simulink model "node23_case_10kV_withLoad_v2"  (R2022b)
settings: Solver=VariableStepAuto  StartTime=0.0  StopTime=10  FixedStep=1e-6  RelTol=1e-5
InitFcn:
  | sw=5;
  | Lf=1.75e-3+3.5e-3;
  | %Lf=3.5e-3;
  | %Cf=2e-4;
  | f=10;
  | Cf=15e-6;
  | % L=1.75e-3/2;
  | % X=100*pi*L;
  | % R=2*X;
  | R=0.25;X=R/0.66;
  | L=X/100/pi;
  | Z=sqrt(R^2+X^2);
  | f = 30;
  | kp1=10;
  | ki1=100;
  | kp4=20;
  | ki4=100;
  | kp16=20;
  | ki16=100;
  | % 负载参数
  | R1L=0;
  | X1L=0;
  | R2L=652.4467;
  | X2L=276.0351;
  | R3L=804.5741;
  | X3L=256.7790;
  | R4L=760.9867;
  | X4L=234.6376;
  | R5L=818.7384;
  | X5L=266.9799;
  | R6L=671.1329;
  | X6L=170.1801;
  | R7L=883.7621;
  | X7L=178.8663;
  | R8L=388.3725;
  | X8L=158.3040;
  | R9L=817.4819;
  | X9L=268.6933;
  | R10L=849.4733;
  | X10L=254.8420;
  | R11L=407.8415;
  | X11L=165.8504;
  | R12L=NaN;  % Bus 12 无 R、X 数据，用 NaN 标记
  | X12L=NaN;
  | R13L=751.2339;
  | X13L=329.8428;
  | R14L=294.0393;
  | X14L=141.6929;
  | R15L=761.9027;
  | X15L=284.3908;
  | R16L=740.4040;
  | X16L=318.2438;
  | R17L=674.5784;
  | X17L=316.4689;
  | R18L=776.7449;
  | X18L=316.6080;
  | R19L=766.0423;
  | X19L=335.7994;
  | R20L=746.0545;
  | X20L=344.3329;
  | ... (+266 lines)
libraries: spsSeriesRLCBranchLib x210, slpidlib x45, spsControlledVoltageSourceLib x30, spsThreePhaseVIMeasurementLib x24, spsPower3phInstantaneousLib x13, spsAlphaBetaZerotoabcLib x9, spsCurrentMeasurementLib x6, spsGroundLib x2, spspowerguiLib x1
(part 6 of 8)

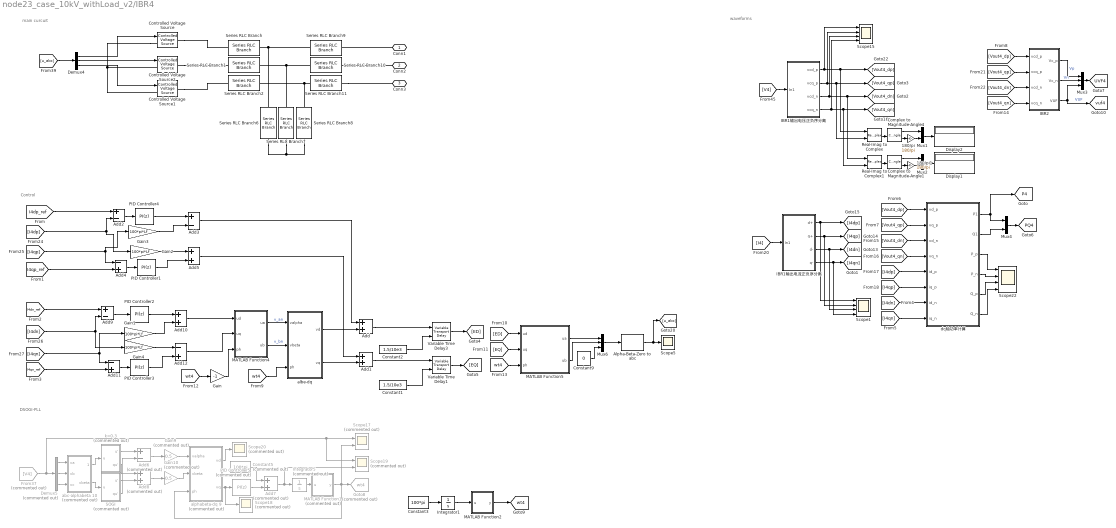
== system node23_case_10kV_withLoad_v2/IBR4 ==
  note: waveforms
  note: Control
  note: main curcuit
  note: DSOGI-PLL
  180/pi : Gain  Gain=180/pi
  180/pi1 : Gain  Gain=180/pi
  Add{,1,5,10} (4 alike) : Sum
  Add11 : Sum  Inputs=-+
  Add12 : Sum  Inputs=-+
  Add2 : Sum  Inputs=+-
  Add3 : Sum  Inputs=+-
  Add4 : Sum  Inputs=-+
  Add6 : Sum  Commented=on  Inputs=+-
  Add7 : Sum  Commented=on
  Add8 : Sum  Commented=on
  Add9 : Sum  Inputs=+-
  Alpha-Beta-Zero to abc : spsAlphaBetaZerotoabcLib/Alpha-Beta-Zero to abc
      settings: LibrarySourceBlock=|
      | sps_lib/Control/Alpha-Beta-Zero
      | to abc
  Complex to Magnitude-Angle1 : ComplexToMagnitudeAngle
  Complex to Magnitude-Angle4 : ComplexToMagnitudeAngle
  Constant1 : Constant  Value=1.5/10e3
  Constant2 : Constant  Value=1.5/10e3
  Constant3 : Constant  Value=100*pi
  Constant5 : Constant  Commented=on  Value=100*pi
  Constant9 : Constant  Value=0
  Controlled Voltage Source : spsControlledVoltageSourceLib/Controlled Voltage Source  Initialize=on  Source_Type=AC  Amplitude=0  Phase=0  Frequency=0  Measurements=None
  Controlled Voltage Source1 : spsControlledVoltageSourceLib/Controlled Voltage Source  Initialize=on  Source_Type=AC  Amplitude=0  Phase=0  Frequency=0  Measurements=None
  Controlled Voltage Source2 : spsControlledVoltageSourceLib/Controlled Voltage Source  Initialize=on  Source_Type=AC  Amplitude=0  Phase=0  Frequency=0  Measurements=None
  Demux4 : Demux  Outputs=3
  Demux5 : Demux  Commented=on  Outputs=3
  Display1 : Display
  Display2 : Display
  From37 : From  Commented=on  GotoTag=V4  TagVisibility=global
  Gain : Gain  Gain=-1
  Gain{1..4} (4 alike) : Gain  Gain=100*pi*Lf
  Gain10 : Gain  Commented=on  Gain=0.5
  Gain9 : Gain  Commented=on  Gain=0.5
  Goto8 : Goto  Commented=on  GotoTag=wt4  TagVisibility=global
  IBR1输出电压正负序分离 : Subsystem
  IBR1输出电流正负序分离 : Subsystem
  IBR2 : MATLAB Function  TreatAsAtomicUnit=on
  Integrator1 : Integrator
  Integrator5 : Integrator  Commented=on
  MATLAB Function1 : MATLAB Function  Commented=on  TreatAsAtomicUnit=on
  MATLAB Function2 : MATLAB Function  TreatAsAtomicUnit=on
  MATLAB Function4 : MATLAB Function  TreatAsAtomicUnit=on
  MATLAB Function5 : MATLAB Function  TreatAsAtomicUnit=on
  Mux1 : Mux  Inputs=2
  Mux2 : Mux  Inputs=2
  Mux3 : Mux  Inputs=3
  Mux4 : Mux  Inputs=2
  Mux6 : Mux  Inputs=3
  PID Controller{1..4} (4 alike) : slpidlib/PID Controller  Controller=PI  Form=Parallel  TimeDomain=Discrete-time  UseExternalTs=off  SampleTime=-1  IntegratorMethod=Forward Euler  FilterMethod=Forward Euler  ControllerParametersSource=internal  P=kp4  I=ki4  UseKiTs=off  D=0  N=100  UseFilter=on  TunerSelectOption=Transfer Function Based (PID Tuner App)  InitialConditionSource=internal  InitialConditionForIntegrator=0  InitialConditionForFilter=0  DifferentiatorICPrevScaledInput=0  ExternalReset=none  TrackingMode=off  Kt=1  LimitOutput=off  SatLimitsSource=internal  UpperSaturationLimit=5  LowerSaturationLimit=-5  LinearizeAsGain=on  AntiWindupMode=none  Kb=1  LimitIntegrator=off  UpperIntegratorSaturationLimit=inf  LowerIntegratorSaturationLimit=-inf  POutMin=[]  POutMax=[]  IOutMin=[]  IOutMax=[]  DOutMin=[]  DOutMax=[]  NOutMin=[]  NOutMax=[]  SumOutMin=[]  SumOutMax=[]  SaturationOutMin=[]  SaturationOutMax=[]  PParamMin=[]  PParamMax=[]  IParamMin=[]  IParamMax=[]  DParamMin=[]  DParamMax=[]  NParamMin=[]  NParamMax=[]  KbParamMin=[]  KbParamMax=[]  KtParamMin=[]  KtParamMax=[]  KbOutMin=[]  KbOutMax=[]  KtOutMin=[]  KtOutMax=[]  IntegratorOutMin=[]  IntegratorOutMax=[]  FilterOutMin=[]  FilterOutMax=[]  SumI1OutMin=[]  SumI1OutMax=[]  SumI2OutMin=[]  SumI2OutMax=[]  SumI3OutMin=[]  SumI3OutMax=[]  SumI4OutMin=[]  SumI4OutMax=[]  SumDOutMin=[]  SumDOutMax=[]  DifferentiatorOutMin=[]  DifferentiatorOutMax=[]  FilterDiffOutCoefMin=[]  FilterDiffOutCoefMax=[]  ReciprocalOutMin=[]  ReciprocalOutMax=[]  SumDenOutMin=[]  SumDenOutMax=[]  SumNumOutMin=[]  SumNumOutMax=[]  DivideOutMin=[]  DivideOutMax=[]  UdiffTsProdOutMin=[]  UdiffTsProdOutMax=[]  NTsProdOutMin=[]  NTsProdOutMax=[]  UintegralTsProdOutMin=[]  UintegralTsProdOutMax=[]  UngainTsProdOutMin=[]  UngainTsProdOutMax=[]  ClampingZeroOutDataTypeStr=Inherit: Inherit via back propagation  ClampingZeroOutMin=[]  ClampingZeroOutMax=[]  FilterDenConstantOutDataTypeStr=Inherit: Inherit via back propagation  FilterDenConstantOutMin=[]  FilterDenConstantOutMax=[]  PCopyOutDataTypeStr=Inherit: Inherit via back propagation  PCopyOutMin=[]  PCopyOutMax=[]  NCopyOutDataTypeStr=Inherit: Inherit via back propagation  NCopyOutMin=[]  NCopyOutMax=[]  IntegratorContinuousStateAttributes=''  IntegratorStateMustResolveToSignalObject=off  IntegratorRTWStateStorageClass=Auto  FilterContinuousStateAttributes=''  FilterStateMustResolveToSignalObject=off  FilterRTWStateStorageClass=Auto  ParallelPVariant=InternalParameters  IdealPVariant=Disabled  IVariant=InternalParameters  DVariant=Disabled  IntegratorVariant=Discrete  SatVariant=Disabled  AWVariant=Passthrough  PCopyVariant=Disabled  TRVariant=Disabled  FdbkBlocksVariant=Forward  IdealPFdbkVariant=Disabled  SatFdbkVariant=Disabled  DerivativeFilterVariant=Disabled  NVariant=Disabled  NCopyVariant=Disabled_SignalSpec  FilterICVariant=Disabled  IntegratorICVariant=InternalICs  ExternalResetVariant=Disabled  TRSumVariant=Passthrough  SumFdbkVariant=Disabled  SumVariant=Sum_PI  TsampFilterVariant=InternalTs  TsampNgainVariant=Passthrough  TsampIntegralVariant=Passthrough  ExternalSaturationOutDataTypeStr=Inherit: Same as second input
  PID Controller5 : slpidlib/PID Controller  Commented=on  Controller=PI  Form=Parallel  TimeDomain=Discrete-time  UseExternalTs=off  SampleTime=-1  IntegratorMethod=Forward Euler  FilterMethod=Forward Euler  ControllerParametersSource=internal  P=1  I=3  UseKiTs=off  D=0  N=100  UseFilter=on  TunerSelectOption=Transfer Function Based (PID Tuner App)  InitialConditionSource=internal  InitialConditionForIntegrator=0  InitialConditionForFilter=0  DifferentiatorICPrevScaledInput=0  ExternalReset=none  TrackingMode=off  Kt=1  LimitOutput=off  SatLimitsSource=internal  UpperSaturationLimit=inf  LowerSaturationLimit=-inf  LinearizeAsGain=on  AntiWindupMode=none  Kb=1  LimitIntegrator=off  UpperIntegratorSaturationLimit=inf  LowerIntegratorSaturationLimit=-inf  POutMin=[]  POutMax=[]  IOutMin=[]  IOutMax=[]  DOutMin=[]  DOutMax=[]  NOutMin=[]  NOutMax=[]  SumOutMin=[]  SumOutMax=[]  SaturationOutMin=[]  SaturationOutMax=[]  PParamMin=[]  PParamMax=[]  IParamMin=[]  IParamMax=[]  DParamMin=[]  DParamMax=[]  NParamMin=[]  NParamMax=[]  KbParamMin=[]  KbParamMax=[]  KtParamMin=[]  KtParamMax=[]  KbOutMin=[]  KbOutMax=[]  KtOutMin=[]  KtOutMax=[]  IntegratorOutMin=[]  IntegratorOutMax=[]  FilterOutMin=[]  FilterOutMax=[]  SumI1OutMin=[]  SumI1OutMax=[]  SumI2OutMin=[]  SumI2OutMax=[]  SumI3OutMin=[]  SumI3OutMax=[]  SumI4OutMin=[]  SumI4OutMax=[]  SumDOutMin=[]  SumDOutMax=[]  DifferentiatorOutMin=[]  DifferentiatorOutMax=[]  FilterDiffOutCoefMin=[]  FilterDiffOutCoefMax=[]  ReciprocalOutMin=[]  ReciprocalOutMax=[]  SumDenOutMin=[]  SumDenOutMax=[]  SumNumOutMin=[]  SumNumOutMax=[]  DivideOutMin=[]  DivideOutMax=[]  UdiffTsProdOutMin=[]  UdiffTsProdOutMax=[]  NTsProdOutMin=[]  NTsProdOutMax=[]  UintegralTsProdOutMin=[]  UintegralTsProdOutMax=[]  UngainTsProdOutMin=[]  UngainTsProdOutMax=[]  ClampingZeroOutDataTypeStr=Inherit: Inherit via back propagation  ClampingZeroOutMin=[]  ClampingZeroOutMax=[]  FilterDenConstantOutDataTypeStr=Inherit: Inherit via back propagation  FilterDenConstantOutMin=[]  FilterDenConstantOutMax=[]  PCopyOutDataTypeStr=Inherit: Inherit via back propagation  PCopyOutMin=[]  PCopyOutMax=[]  NCopyOutDataTypeStr=Inherit: Inherit via back propagation  NCopyOutMin=[]  NCopyOutMax=[]  IntegratorContinuousStateAttributes=''  IntegratorStateMustResolveToSignalObject=off  IntegratorRTWStateStorageClass=Auto  FilterContinuousStateAttributes=''  FilterStateMustResolveToSignalObject=off  FilterRTWStateStorageClass=Auto  ParallelPVariant=InternalParameters  IdealPVariant=Disabled  IVariant=InternalParameters  DVariant=Disabled  IntegratorVariant=Discrete  SatVariant=Disabled  AWVariant=Passthrough  PCopyVariant=Disabled  TRVariant=Disabled  FdbkBlocksVariant=Forward  IdealPFdbkVariant=Disabled  SatFdbkVariant=Disabled  DerivativeFilterVariant=Disabled  NVariant=Disabled  NCopyVariant=Disabled_SignalSpec  FilterICVariant=Disabled  IntegratorICVariant=InternalICs  ExternalResetVariant=Disabled  TRSumVariant=Passthrough  SumFdbkVariant=Disabled  SumVariant=Sum_PI  TsampFilterVariant=InternalTs  TsampNgainVariant=Passthrough  TsampIntegralVariant=Passthrough  ExternalSaturationOutDataTypeStr=Inherit: Same as second input
  Real-Imag to Complex : RealImagToComplex
  Real-Imag to Complex1 : RealImagToComplex
  SOGI : Subsystem  Commented=on
  Scope1 : Scope  NumInputPorts=4
  Scope15 : Scope  NumInputPorts=4
  Scope17 : Scope  Commented=on  NumInputPorts=2
  Scope18 : Scope  Commented=on
  Scope19 : Scope  Commented=on  NumInputPorts=2
  Scope20 : Scope  Commented=on
  Scope22 : Scope  NumInputPorts=4
  Scope5 : Scope
  Series RLC Branch : spsSeriesRLCBranchLib/Series RLC Branch  LConnTagsString=__new0  RConnTagsString=__new0  BranchType=L  Resistance=1  Inductance=3.5e-3  SetiL0=off  InitialCurrent=0  Capacitance=1e-6  Setx0=off  InitialVoltage=0  Measurements=None
  Series RLC Branch1 : spsSeriesRLCBranchLib/Series RLC Branch  LConnTagsString=__new0  RConnTagsString=__new0  BranchType=L  Resistance=1  Inductance=3.5e-3  SetiL0=off  InitialCurrent=0  Capacitance=1e-6  Setx0=off  InitialVoltage=0  Measurements=None
  Series RLC Branch10 : spsSeriesRLCBranchLib/Series RLC Branch  LConnTagsString=__new0  RConnTagsString=__new0  BranchType=L  Resistance=1  Inductance=1.75e-3  SetiL0=off  InitialCurrent=0  Capacitance=1e-6  Setx0=off  InitialVoltage=0  Measurements=None
  Series RLC Branch11 : spsSeriesRLCBranchLib/Series RLC Branch  LConnTagsString=__new0  RConnTagsString=__new0  BranchType=L  Resistance=1  Inductance=1.75e-3  SetiL0=off  InitialCurrent=0  Capacitance=1e-6  Setx0=off  InitialVoltage=0  Measurements=None
  Series RLC Branch2 : spsSeriesRLCBranchLib/Series RLC Branch  LConnTagsString=__new0  RConnTagsString=__new0  BranchType=L  Resistance=1  Inductance=3.5e-3  SetiL0=off  InitialCurrent=0  Capacitance=1e-6  Setx0=off  InitialVoltage=0  Measurements=None
  Series RLC Branch6 : spsSeriesRLCBranchLib/Series RLC Branch  LConnTagsString=__new0  RConnTagsString=__new0  BranchType=RC  Resistance=5  Inductance=500e-6  SetiL0=off  InitialCurrent=0  Capacitance=Cf  Setx0=off  InitialVoltage=0  Measurements=None
  Series RLC Branch7 : spsSeriesRLCBranchLib/Series RLC Branch  LConnTagsString=__new0  RConnTagsString=__new0  BranchType=RC  Resistance=5  Inductance=500e-6  SetiL0=off  InitialCurrent=0  Capacitance=Cf  Setx0=off  InitialVoltage=0  Measurements=None
  Series RLC Branch8 : spsSeriesRLCBranchLib/Series RLC Branch  LConnTagsString=__new0  RConnTagsString=__new0  BranchType=RC  Resistance=5  Inductance=500e-6  SetiL0=off  InitialCurrent=0  Capacitance=Cf  Setx0=off  InitialVoltage=0  Measurements=None
  Series RLC Branch9 : spsSeriesRLCBranchLib/Series RLC Branch  LConnTagsString=__new0  RConnTagsString=__new0  BranchType=L  Resistance=1  Inductance=1.75e-3  SetiL0=off  InitialCurrent=0  Capacitance=1e-6  Setx0=off  InitialVoltage=0  Measurements=None
  Variable Time Delay1 : VariableTransportDelay  MaximumDelay=10  PadeOrder=2
  Variable Time Delay3 : VariableTransportDelay  MaximumDelay=10  PadeOrder=2
  abc-alphabeta 10 : MATLAB Function  Commented=on  TreatAsAtomicUnit=on
  albe-dq : MATLAB Function  TreatAsAtomicUnit=on
  alphabeta-dq 9 : MATLAB Function  Commented=on  TreatAsAtomicUnit=on
  dq轴功率计算 : MATLAB Function  TreatAsAtomicUnit=on
  k=0.3 : Subsystem  Commented=on
  Conn1 : PMIOPort  Side=Right
  Conn2 : PMIOPort  Port=2  Side=Right
  Conn3 : PMIOPort  Port=3  Side=Right
  tag scope: P4=global, PQ4=global, UVF4=global, vuf4=global, wt4=global
  wires:
  [EQ] -> MATLAB Function5/2(uq)
  Add12/1 -> MATLAB Function4/2(uq)
  [wt4] -> MATLAB Function5/3(ph)
  Add3/1 -> Add/1
  PID Controller3/1 -> Add12/2
  PID Controller2/1 -> Add10/1
  [I4dp] -> Gain2/1, Add2/2
  Gain4/1 -> Add12/1
  Gain/1 -> MATLAB Function4/3(ph)
  Add9/1 -> PID Controller2/1
  MATLAB Function5/2(ub) -> Mux6/2
  MATLAB Function4/2(ub) -> albe-dq/2(vbeta)  "v_bn"
  Add2/1 -> PID Controller4/1
  Add10/1 -> MATLAB Function4/1(ud)
  Add11/1 -> PID Controller3/1
  [ED] -> MATLAB Function5/1(ud)
  Add4/1 -> PID Controller1/1
  Gain3/1 -> Add3/2
  PID Controller4/1 -> Add3/1
  [wt4] -> albe-dq/3(ph)
  [I4qp] -> Add4/1, Gain3/1
  Gain2/1 -> Add5/1
  albe-dq/1(vd) -> Add/2
  Add5/1 -> Add1/1
  Gain1/1 -> Add10/2
  albe-dq/2(vq) -> Add1/2
  PID Controller1/1 -> Add5/2
  [I4dn] -> Gain4/1, Add9/2
  [I4qn] -> Gain1/1, Add11/1
  MATLAB Function4/1(ua) -> albe-dq/1(valpha)  "v_an"
  [wt4] -> Gain/1
  Demux4/3 -> Controlled Voltage Source1/1
  Demux4/2 -> Controlled Voltage Source2/1
  Demux4/1 -> Controlled Voltage Source/1
  [u_abc] -> Demux4/1
  Mux6/1 -> Alpha-Beta-Zero to abc/1
  Alpha-Beta-Zero to abc/1 -> [u_abc], Scope5/1
  Constant9/1 -> Mux6/3
  MATLAB Function5/1(ua) -> Mux6/1
  [I4dp_ref] -> Add2/1
  [I4qp_ref] -> Add4/2
  [I4dn_ref] -> Add9/1
  [I4qn_ref] -> Add11/2
  Complex to Magnitude-Angle4/2 -> 180/pi/1
  IBR1输出电压正负序分离/4(vcq_n) -> Scope15/4, Real-Imag to Complex1/2, [Vout4_qn]
  IBR2/1(Vc_p) -> Mux3/1  "Vp"
  IBR1输出电流正负序分离/3(d-) -> Scope1/3, [I4dn]
  dq轴功率计算/3(P_p) -> Scope22/1
  dq轴功率计算/1(P1) -> Mux4/1, [P4]
  Real-Imag to Complex1/1 -> Complex to Magnitude-Angle1/1
  [I4qn] -> dq轴功率计算/8(iq_n)
  [Vout4_dp] -> dq轴功率计算/1(vd_p)
  [Vout4_qp] -> dq轴功率计算/2(vq_p)
  [I4dp] -> dq轴功率计算/5(id_p)
  [I4] -> IBR1输出电流正负序分离/1(In1)
  dq轴功率计算/5(Q_p) -> Scope22/3
  [I4dn] -> dq轴功率计算/7(id_n)
  [I4qp] -> dq轴功率计算/6(iq_p)
  dq轴功率计算/2(Q1) -> Mux4/2
  [Vout4_dp] -> IBR2/1(vcd_p)
  IBR1输出电流正负序分离/4(q-) -> Scope1/4, [I4qn]
  [Vout4_qp] -> IBR2/2(vcq_p)
  [Vout4_dn] -> IBR2/3(vcd_n)
  IBR1输出电流正负序分离/2(q+) -> [I4qp], Scope1/2
  180/pi/1 -> Mux1/2
  Real-Imag to Complex/1 -> Complex to Magnitude-Angle4/1
  [V4] -> IBR1输出电压正负序分离/1(In1)
  [Vout4_qn] -> IBR2/4(vcq_n)
  180/pi1/1 -> Mux2/2
  IBR1输出电压正负序分离/1(vcd_p) -> [Vout4_dp], Real-Imag to Complex/1, Scope15/1
  Complex to Magnitude-Angle1/2 -> 180/pi1/1
  Mux4/1 -> [PQ4]
  Mux2/1 -> Display1/1
  Complex to Magnitude-Angle1/1 -> Mux2/1
  IBR2/2(Vc_n) -> Mux3/2  "Vn"
  [Vout4_qn] -> dq轴功率计算/4(vq_n)
  IBR1输出电压正负序分离/3(vcd_n) -> Real-Imag to Complex1/1, [Vout4_dn], Scope15/3
  IBR1输出电压正负序分离/2(vcq_p) -> Real-Imag to Complex/2, [Vout4_qp], Scope15/2
  dq轴功率计算/6(Q_n) -> Scope22/4
  Mux1/1 -> Display2/1
  dq轴功率计算/4(P_n) -> Scope22/2
  Complex to Magnitude-Angle4/1 -> Mux1/1
  [Vout4_dn] -> dq轴功率计算/3(vd_n)
  IBR2/3(VUF) -> [vuf4], Mux3/3  "VUF"
  Mux3/1 -> [UVF4]
  Variable Time Delay1/1 -> [EQ]
  Constant1/1 -> Variable Time Delay1/2
  Add/1 -> Variable Time Delay3/1
  Add1/1 -> Variable Time Delay1/1
  Constant2/1 -> Variable Time Delay3/2
  Variable Time Delay3/1 -> [ED]
  SOGI/2(qu') -> Add6/2
  Demux5/1 -> abc-alphabeta 10/1(va)
  Demux5/3 -> abc-alphabeta 10/3(vc)
  PID Controller5/1 -> Add7/2
  k=0.3/2(qu') -> Add8/1
  k=0.3/1(u') -> Add6/1
  abc-alphabeta 10/2(vbeta) -> SOGI/1(u)
  abc-alphabeta 10/1(valpha) -> k=0.3/1(u)
  From37/1 -> Scope19/1, Scope17/1, Demux5/1
  Add6/1 -> Gain9/1
  alphabeta-dq 9/2(vq) -> Scope18/1, PID Controller5/1
  Demux5/2 -> abc-alphabeta 10/2(vb)
  Gain10/1 -> alphabeta-dq 9/2(vbeta)
  SOGI/1(u') -> Add8/2
  Add7/1 -> Integrator5/1, Scope19/2
  MATLAB Function1/1(y) -> Goto8/1, Scope17/2, alphabeta-dq 9/3(ph)
  alphabeta-dq 9/1(vd) -> Scope20/1
  Add8/1 -> Gain10/1
  Integrator5/1 -> MATLAB Function1/1(u)
  Gain9/1 -> alphabeta-dq 9/1(valpha)
  Constant5/1 -> Add7/1
  Integrator1/1 -> MATLAB Function2/1(u)
  Constant3/1 -> Integrator1/1
  MATLAB Function2/1(y) -> [wt4]
  IBR1输出电流正负序分离/1(d+) -> [I4dp], Scope1/1
  connections:
  Series RLC Branch11/LConn1 -- Series RLC Branch2/RConn1 -- Series RLC Branch8/LConn1
  Series RLC Branch10/LConn1 -- Series RLC Branch7/LConn1 -- Series RLC Branch1/RConn1
  Series RLC Branch9/LConn1 -- Series RLC Branch6/LConn1 -- Series RLC Branch/RConn1
  Controlled Voltage Source2/RConn1 -- Series RLC Branch1/LConn1
  Controlled Voltage Source1/RConn1 -- Series RLC Branch2/LConn1
  Series RLC Branch7/RConn1 -- Series RLC Branch6/RConn1 -- Series RLC Branch8/RConn1
  Controlled Voltage Source/RConn1 -- Series RLC Branch/LConn1
  Series RLC Branch11/RConn1 -- Conn3/RConn1
  Series RLC Branch10/RConn1 -- Conn2/RConn1
  Conn1/RConn1 -- Series RLC Branch9/RConn1
  Controlled Voltage Source/LConn1 -- Controlled Voltage Source2/LConn1 -- Controlled Voltage Source1/LConn1

== system node23_case_10kV_withLoad_v2/Subsystem1 ==
  Current : spsCurrentMeasurementLib/Current Measurement  PhasorSimulation=off  OutputType=Complex  PSBequivalent=0
  Current 2 : spsCurrentMeasurementLib/Current Measurement  PhasorSimulation=off  OutputType=Complex  PSBequivalent=0
  Current1 : spsCurrentMeasurementLib/Current Measurement  PhasorSimulation=off  OutputType=Complex  PSBequivalent=0
  1 : PMIOPort  Side=Left
  3 : PMIOPort  Port=2  Side=Left
  5 : PMIOPort  Port=3  Side=Left
  2 : PMIOPort  Port=4  Side=Right
  4 : PMIOPort  Port=5  Side=Right
  6 : PMIOPort  Port=6  Side=Right
  O1 : Outport
  O2 : Outport  Port=2
  O3 : Outport  Port=3
  wires:
  Current/1 -> O1/1
  Current1/1 -> O2/1
  Current 2/1 -> O3/1
  connections:
  1/RConn1 -- Current/LConn1
  2/RConn1 -- Current/RConn1
  3/RConn1 -- Current1/LConn1
  4/RConn1 -- Current1/RConn1
  5/RConn1 -- Current 2/LConn1
  6/RConn1 -- Current 2/RConn1

== system node23_case_10kV_withLoad_v2/Subsystem10 ==
  Current : spsCurrentMeasurementLib/Current Measurement  PhasorSimulation=off  OutputType=Complex  PSBequivalent=0
  Current 2 : spsCurrentMeasurementLib/Current Measurement  PhasorSimulation=off  OutputType=Complex  PSBequivalent=0
  Current1 : spsCurrentMeasurementLib/Current Measurement  PhasorSimulation=off  OutputType=Complex  PSBequivalent=0
  1 : PMIOPort  Side=Left
  3 : PMIOPort  Port=2  Side=Left
  5 : PMIOPort  Port=3  Side=Left
  2 : PMIOPort  Port=4  Side=Right
  4 : PMIOPort  Port=5  Side=Right
  6 : PMIOPort  Port=6  Side=Right
  O1 : Outport
  O2 : Outport  Port=2
  O3 : Outport  Port=3
  wires:
  Current 2/1 -> O3/1
  Current1/1 -> O2/1
  Current/1 -> O1/1
  connections:
  6/RConn1 -- Current 2/RConn1
  5/RConn1 -- Current 2/LConn1
  4/RConn1 -- Current1/RConn1
  3/RConn1 -- Current1/LConn1
  2/RConn1 -- Current/RConn1
  1/RConn1 -- Current/LConn1

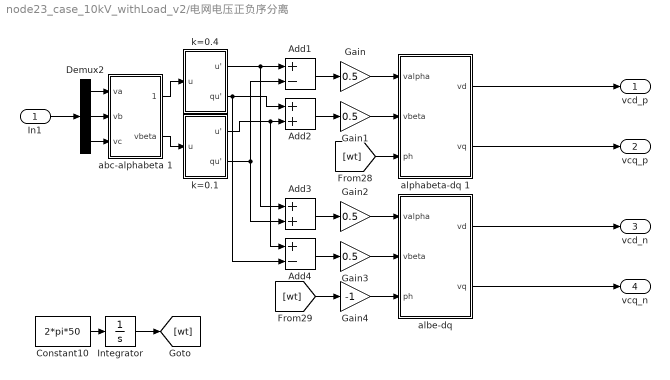
== system node23_case_10kV_withLoad_v2/电网电压正负序分离 ==
  In1 : Inport
  Add1 : Sum  Inputs=+-
  Add2 : Sum
  Add3 : Sum
  Add4 : Sum  Inputs=+-
  Constant10 : Constant  Value=2*pi*50
  Demux2 : Demux  Outputs=3
  Gain{,1..3} (4 alike) : Gain  Gain=0.5
  Gain4 : Gain  Gain=-1
  Integrator : Integrator
  abc-alphabeta 1 : MATLAB Function  TreatAsAtomicUnit=on
  albe-dq : MATLAB Function  TreatAsAtomicUnit=on
  alphabeta-dq 1 : MATLAB Function  TreatAsAtomicUnit=on
  k=0.1 : Subsystem
  k=0.4 : Subsystem
  vcd_p : Outport  VectorParamsAs1DForOutWhenUnconnected=off
  vcq_p : Outport  Port=2  VectorParamsAs1DForOutWhenUnconnected=off
  vcd_n : Outport  Port=3  VectorParamsAs1DForOutWhenUnconnected=off
  vcq_n : Outport  Port=4  VectorParamsAs1DForOutWhenUnconnected=off
  wires:
  abc-alphabeta 1/1(valpha) -> k=0.4/1(u)
  Gain3/1 -> albe-dq/2(vbeta)
  abc-alphabeta 1/2(vbeta) -> k=0.1/1(u)
  Add4/1 -> Gain3/1
  albe-dq/2(vq) -> vcq_n/1
  Gain4/1 -> albe-dq/3(ph)
  [wt] -> alphabeta-dq 1/3(ph)
  Demux2/3 -> abc-alphabeta 1/3(vc)
  alphabeta-dq 1/2(vq) -> vcq_p/1
  Gain2/1 -> albe-dq/1(valpha)
  In1/1 -> Demux2/1
  Gain1/1 -> alphabeta-dq 1/2(vbeta)
  [wt] -> Gain4/1
  Add3/1 -> Gain2/1
  alphabeta-dq 1/1(vd) -> vcd_p/1
  Add2/1 -> Gain1/1
  k=0.1/2(qu') -> Add3/2, Add1/2
  albe-dq/1(vd) -> vcd_n/1
  k=0.4/2(qu') -> Add4/2, Add2/1
  Gain/1 -> alphabeta-dq 1/1(valpha)
  Demux2/1 -> abc-alphabeta 1/1(va)
  Add1/1 -> Gain/1
  k=0.1/1(u') -> Add2/2, Add4/1
  k=0.4/1(u') -> Add1/1, Add3/1
  Demux2/2 -> abc-alphabeta 1/2(vb)
  Constant10/1 -> Integrator/1
  Integrator/1 -> [wt]

== system node23_case_10kV_withLoad_v2/Grid/negative_sequence_dq>>abc4 ==
  note: alpha_beta_0
  note: 0
  note: q
  note: d
  dq0 : Inport
  theta : Inport  Port=2
  Demux3 : Demux  Outputs=3
      settings: DisplayOption=none
  MATLAB Function : MATLAB Function  TreatAsAtomicUnit=on
  Mux1 : Mux  Inputs=3
  dq0>>alpha_beta_0 : Subsystem
  abc : Outport
  wires:
  theta/1 -> MATLAB Function/3(theta)
  Demux3/3 -> Mux1/3
  MATLAB Function/2(beta) -> Mux1/2
  MATLAB Function/1(alpha) -> Mux1/1
  Demux3/2 -> MATLAB Function/2(q)
  Demux3/1 -> MATLAB Function/1(d)
  dq0>>alpha_beta_0/1(abc) -> abc/1
  Mux1/1 -> dq0>>alpha_beta_0/1(alpha_beta_0)
  dq0/1 -> Demux3/1

== system node23_case_10kV_withLoad_v2/Grid/positive_sequence_dq>>abc1 ==
  note: alpha axis 与A axis 重合
  note: alpha_beta_0
  note: 0
  note: q
  note: d
  dq0 : Inport
  theta : Inport  Port=2
  Demux3 : Demux  Outputs=3
      settings: DisplayOption=none
  MATLAB Function : MATLAB Function  TreatAsAtomicUnit=on
  Mux1 : Mux  Inputs=3
  dq0>>alpha_beta_0 : Subsystem
  abc : Outport
  wires:
  theta/1 -> MATLAB Function/3(theta)
  Demux3/3 -> Mux1/3
  MATLAB Function/2(beta) -> Mux1/2
  MATLAB Function/1(alpha) -> Mux1/1
  Demux3/2 -> MATLAB Function/2(q)
  Demux3/1 -> MATLAB Function/1(d)
  dq0>>alpha_beta_0/1(abc) -> abc/1
  Mux1/1 -> dq0>>alpha_beta_0/1(alpha_beta_0)
  dq0/1 -> Demux3/1

== system node23_case_10kV_withLoad_v2/IBR-10/IBR1输出电压正负序分离 ==
  In1 : Inport
  Add1 : Sum  Inputs=+-
  Add2 : Sum
  Add3 : Sum
  Add4 : Sum  Inputs=+-
  Demux2 : Demux  Outputs=3
  Gain{,1..3} (4 alike) : Gain  Gain=0.5
  Gain4 : Gain  Gain=-1
  abc-alphabeta 1 : MATLAB Function  TreatAsAtomicUnit=on
  albe-dq : MATLAB Function  TreatAsAtomicUnit=on
  alphabeta-dq 1 : MATLAB Function  TreatAsAtomicUnit=on
  k=0.1 : Subsystem
  k=0.4 : Subsystem
  vcd_p : Outport  VectorParamsAs1DForOutWhenUnconnected=off
  vcq_p : Outport  Port=2  VectorParamsAs1DForOutWhenUnconnected=off
  vcd_n : Outport  Port=3  VectorParamsAs1DForOutWhenUnconnected=off
  vcq_n : Outport  Port=4  VectorParamsAs1DForOutWhenUnconnected=off
  wires:
  Demux2/2 -> abc-alphabeta 1/2(vb)
  k=0.4/1(u') -> Add3/1, Add1/1
  k=0.1/1(u') -> Add4/1, Add2/2
  Add1/1 -> Gain/1
  Demux2/1 -> abc-alphabeta 1/1(va)
  Gain/1 -> alphabeta-dq 1/1(valpha)
  k=0.4/2(qu') -> Add2/1, Add4/2
  albe-dq/1(vd) -> vcd_n/1
  k=0.1/2(qu') -> Add1/2, Add3/2
  Add2/1 -> Gain1/1
  alphabeta-dq 1/1(vd) -> vcd_p/1
  Add3/1 -> Gain2/1
  [wt10] -> Gain4/1
  Gain1/1 -> alphabeta-dq 1/2(vbeta)
  In1/1 -> Demux2/1
  Gain2/1 -> albe-dq/1(valpha)
  alphabeta-dq 1/2(vq) -> vcq_p/1
  Demux2/3 -> abc-alphabeta 1/3(vc)
  [wt10] -> alphabeta-dq 1/3(ph)
  Gain4/1 -> albe-dq/3(ph)
  albe-dq/2(vq) -> vcq_n/1
  Add4/1 -> Gain3/1
  abc-alphabeta 1/2(vbeta) -> k=0.1/1(u)
  Gain3/1 -> albe-dq/2(vbeta)
  abc-alphabeta 1/1(valpha) -> k=0.4/1(u)

== system node23_case_10kV_withLoad_v2/IBR-10/IBR1输出电流正负序分离 ==
  In1 : Inport
  Add1 : Sum  Inputs=+-
  Add2 : Sum
  Add3 : Sum
  Add4 : Sum  Inputs=+-
  Demux2 : Demux  Outputs=3
  Gain{,1..3} (4 alike) : Gain  Gain=0.5
  Gain4 : Gain  Gain=-1
  abc-alphabeta 1 : MATLAB Function  TreatAsAtomicUnit=on
  albe-dq : MATLAB Function  TreatAsAtomicUnit=on
  alphabeta-dq 1 : MATLAB Function  TreatAsAtomicUnit=on
  k=0.1 : Subsystem
  k=0.4 : Subsystem
  d+ : Outport  VectorParamsAs1DForOutWhenUnconnected=off
  q+ : Outport  Port=2  VectorParamsAs1DForOutWhenUnconnected=off
  d- : Outport  Port=3  VectorParamsAs1DForOutWhenUnconnected=off
  q- : Outport  Port=4  VectorParamsAs1DForOutWhenUnconnected=off
  wires:
  albe-dq/2(vq) -> q-/1
  albe-dq/1(vd) -> d-/1
  alphabeta-dq 1/2(vq) -> q+/1
  alphabeta-dq 1/1(vd) -> d+/1
  abc-alphabeta 1/1(valpha) -> k=0.4/1(u)
  Gain3/1 -> albe-dq/2(vbeta)
  abc-alphabeta 1/2(vbeta) -> k=0.1/1(u)
  Add4/1 -> Gain3/1
  Gain4/1 -> albe-dq/3(ph)
  [wt10] -> alphabeta-dq 1/3(ph)
  Demux2/3 -> abc-alphabeta 1/3(vc)
  Gain2/1 -> albe-dq/1(valpha)
  In1/1 -> Demux2/1
  Gain1/1 -> alphabeta-dq 1/2(vbeta)
  [wt10] -> Gain4/1
  Add3/1 -> Gain2/1
  Add2/1 -> Gain1/1
  k=0.1/2(qu') -> Add3/2, Add1/2
  k=0.4/2(qu') -> Add4/2, Add2/1
  Gain/1 -> alphabeta-dq 1/1(valpha)
  Demux2/1 -> abc-alphabeta 1/1(va)
  Add1/1 -> Gain/1
  k=0.1/1(u') -> Add2/2, Add4/1
  k=0.4/1(u') -> Add1/1, Add3/1
  Demux2/2 -> abc-alphabeta 1/2(vb)

== system node23_case_10kV_withLoad_v2/IBR-10/SOGI ==
  u : Inport
  Gain1 : Gain  Gain=314.15926
  Gain2 : Gain  Gain=0.707
  Gain3 : Gain  Gain=314.15926
  Integrator : Integrator
  Integrator1 : Integrator
  Sum : Sum  Inputs=-+|
  Sum1 : Sum  Inputs=|+-
  u' : Outport
  qu' : Outport  Port=2
  wires:
  Gain1/1 -> Integrator/1
  Sum1/1 -> Gain1/1
  u/1 -> Sum/2
  Integrator/1 -> Integrator1/1, u'/1, Sum/1  "u'"
  Gain2/1 -> Sum1/1
  Integrator1/1 -> Gain3/1
  Gain3/1 -> qu'/1, Sum1/2  "qu'"
  Sum/1 -> Gain2/1

== system node23_case_10kV_withLoad_v2/IBR-10/k=0.3 ==
  u : Inport
  Gain1 : Gain  Gain=314.15926
  Gain2 : Gain  Gain=0.707
  Gain3 : Gain  Gain=314.15926
  Integrator : Integrator
  Integrator1 : Integrator
  Sum : Sum  Inputs=-+|
  Sum1 : Sum  Inputs=|+-
  u' : Outport
  qu' : Outport  Port=2
  wires:
  Gain1/1 -> Integrator/1
  Sum1/1 -> Gain1/1
  u/1 -> Sum/2
  Integrator/1 -> Integrator1/1, u'/1, Sum/1  "u'"
  Gain2/1 -> Sum1/1
  Integrator1/1 -> Gain3/1
  Gain3/1 -> qu'/1, Sum1/2  "qu'"
  Sum/1 -> Gain2/1

== system node23_case_10kV_withLoad_v2/IBR-11/IBR1输出电压正负序分离 ==
  In1 : Inport
  Add1 : Sum  Inputs=+-
  Add2 : Sum
  Add3 : Sum
  Add4 : Sum  Inputs=+-
  Demux2 : Demux  Outputs=3
  Gain{,1..3} (4 alike) : Gain  Gain=0.5
  Gain4 : Gain  Gain=-1
  abc-alphabeta 1 : MATLAB Function  TreatAsAtomicUnit=on
  albe-dq : MATLAB Function  TreatAsAtomicUnit=on
  alphabeta-dq 1 : MATLAB Function  TreatAsAtomicUnit=on
  k=0.1 : Subsystem
  k=0.4 : Subsystem
  Out1 : Outport  VectorParamsAs1DForOutWhenUnconnected=off
  Out2 : Outport  Port=2  VectorParamsAs1DForOutWhenUnconnected=off
  Out3 : Outport  Port=3  VectorParamsAs1DForOutWhenUnconnected=off
  Out4 : Outport  Port=4  VectorParamsAs1DForOutWhenUnconnected=off
  wires:
  Demux2/2 -> abc-alphabeta 1/2(vb)
  k=0.4/1(u') -> Add3/1, Add1/1
  k=0.1/1(u') -> Add4/1, Add2/2
  Add1/1 -> Gain/1
  Demux2/1 -> abc-alphabeta 1/1(va)
  Gain/1 -> alphabeta-dq 1/1(valpha)
  k=0.4/2(qu') -> Add2/1, Add4/2
  albe-dq/1(vd) -> Out3/1
  k=0.1/2(qu') -> Add1/2, Add3/2
  Add2/1 -> Gain1/1
  alphabeta-dq 1/1(vd) -> Out1/1
  Add3/1 -> Gain2/1
  [wt11] -> Gain4/1
  Gain1/1 -> alphabeta-dq 1/2(vbeta)
  In1/1 -> Demux2/1
  Gain2/1 -> albe-dq/1(valpha)
  alphabeta-dq 1/2(vq) -> Out2/1
  Demux2/3 -> abc-alphabeta 1/3(vc)
  [wt11] -> alphabeta-dq 1/3(ph)
  Gain4/1 -> albe-dq/3(ph)
  albe-dq/2(vq) -> Out4/1
  Add4/1 -> Gain3/1
  abc-alphabeta 1/2(vbeta) -> k=0.1/1(u)
  Gain3/1 -> albe-dq/2(vbeta)
  abc-alphabeta 1/1(valpha) -> k=0.4/1(u)

== system node23_case_10kV_withLoad_v2/IBR-11/IBR1输出电流正负序分离 ==
  In1 : Inport
  Add1 : Sum  Inputs=+-
  Add2 : Sum
  Add3 : Sum
  Add4 : Sum  Inputs=+-
  Demux2 : Demux  Outputs=3
  Gain{,1..3} (4 alike) : Gain  Gain=0.5
  Gain4 : Gain  Gain=-1
  abc-alphabeta 1 : MATLAB Function  TreatAsAtomicUnit=on
  albe-dq : MATLAB Function  TreatAsAtomicUnit=on
  alphabeta-dq 1 : MATLAB Function  TreatAsAtomicUnit=on
  k=0.1 : Subsystem
  k=0.4 : Subsystem
  d+ : Outport  VectorParamsAs1DForOutWhenUnconnected=off
  q+ : Outport  Port=2  VectorParamsAs1DForOutWhenUnconnected=off
  d- : Outport  Port=3  VectorParamsAs1DForOutWhenUnconnected=off
  q- : Outport  Port=4  VectorParamsAs1DForOutWhenUnconnected=off
  wires:
  albe-dq/2(vq) -> q-/1
  albe-dq/1(vd) -> d-/1
  alphabeta-dq 1/2(vq) -> q+/1
  alphabeta-dq 1/1(vd) -> d+/1
  abc-alphabeta 1/1(valpha) -> k=0.4/1(u)
  Gain3/1 -> albe-dq/2(vbeta)
  abc-alphabeta 1/2(vbeta) -> k=0.1/1(u)
  Add4/1 -> Gain3/1
  Gain4/1 -> albe-dq/3(ph)
  [wt11] -> alphabeta-dq 1/3(ph)
  Demux2/3 -> abc-alphabeta 1/3(vc)
  Gain2/1 -> albe-dq/1(valpha)
  In1/1 -> Demux2/1
  Gain1/1 -> alphabeta-dq 1/2(vbeta)
  [wt11] -> Gain4/1
  Add3/1 -> Gain2/1
  Add2/1 -> Gain1/1
  k=0.1/2(qu') -> Add3/2, Add1/2
  k=0.4/2(qu') -> Add4/2, Add2/1
  Gain/1 -> alphabeta-dq 1/1(valpha)
  Demux2/1 -> abc-alphabeta 1/1(va)
  Add1/1 -> Gain/1
  k=0.1/1(u') -> Add2/2, Add4/1
  k=0.4/1(u') -> Add1/1, Add3/1
  Demux2/2 -> abc-alphabeta 1/2(vb)

== system node23_case_10kV_withLoad_v2/IBR-11/SOGI ==
  u : Inport
  Gain1 : Gain  Gain=314.15926
  Gain2 : Gain  Gain=0.707
  Gain3 : Gain  Gain=314.15926
  Integrator : Integrator
  Integrator1 : Integrator
  Sum : Sum  Inputs=-+|
  Sum1 : Sum  Inputs=|+-
  u' : Outport
  qu' : Outport  Port=2
  wires:
  Sum/1 -> Gain2/1
  Gain3/1 -> Sum1/2, qu'/1  "qu'"
  Integrator1/1 -> Gain3/1
  Gain2/1 -> Sum1/1
  Integrator/1 -> Sum/1, u'/1, Integrator1/1  "u'"
  u/1 -> Sum/2
  Sum1/1 -> Gain1/1
  Gain1/1 -> Integrator/1

== system node23_case_10kV_withLoad_v2/IBR-11/k=0.3 ==
  u : Inport
  Gain1 : Gain  Gain=314.15926
  Gain2 : Gain  Gain=0.707
  Gain3 : Gain  Gain=314.15926
  Integrator : Integrator
  Integrator1 : Integrator
  Sum : Sum  Inputs=-+|
  Sum1 : Sum  Inputs=|+-
  u' : Outport
  qu' : Outport  Port=2
  wires:
  Sum/1 -> Gain2/1
  Gain3/1 -> Sum1/2, qu'/1  "qu'"
  Integrator1/1 -> Gain3/1
  Gain2/1 -> Sum1/1
  Integrator/1 -> Sum/1, u'/1, Integrator1/1  "u'"
  u/1 -> Sum/2
  Sum1/1 -> Gain1/1
  Gain1/1 -> Integrator/1

== system node23_case_10kV_withLoad_v2/IBR-12/IBR1输出电压正负序分离 ==
  In1 : Inport
  Add1 : Sum  Inputs=+-
  Add2 : Sum
  Add3 : Sum
  Add4 : Sum  Inputs=+-
  Demux2 : Demux  Outputs=3
  Gain{,1..3} (4 alike) : Gain  Gain=0.5
  Gain4 : Gain  Gain=-1
  abc-alphabeta 1 : MATLAB Function  TreatAsAtomicUnit=on
  albe-dq : MATLAB Function  TreatAsAtomicUnit=on
  alphabeta-dq 1 : MATLAB Function  TreatAsAtomicUnit=on
  k=0.1 : Subsystem
  k=0.4 : Subsystem
  Out1 : Outport  VectorParamsAs1DForOutWhenUnconnected=off
  Out2 : Outport  Port=2  VectorParamsAs1DForOutWhenUnconnected=off
  Out3 : Outport  Port=3  VectorParamsAs1DForOutWhenUnconnected=off
  Out4 : Outport  Port=4  VectorParamsAs1DForOutWhenUnconnected=off
  wires:
  Demux2/2 -> abc-alphabeta 1/2(vb)
  k=0.4/1(u') -> Add3/1, Add1/1
  k=0.1/1(u') -> Add4/1, Add2/2
  Add1/1 -> Gain/1
  Demux2/1 -> abc-alphabeta 1/1(va)
  Gain/1 -> alphabeta-dq 1/1(valpha)
  k=0.4/2(qu') -> Add2/1, Add4/2
  albe-dq/1(vd) -> Out3/1
  k=0.1/2(qu') -> Add1/2, Add3/2
  Add2/1 -> Gain1/1
  alphabeta-dq 1/1(vd) -> Out1/1
  Add3/1 -> Gain2/1
  [wt12] -> Gain4/1
  Gain1/1 -> alphabeta-dq 1/2(vbeta)
  In1/1 -> Demux2/1
  Gain2/1 -> albe-dq/1(valpha)
  alphabeta-dq 1/2(vq) -> Out2/1
  Demux2/3 -> abc-alphabeta 1/3(vc)
  [wt12] -> alphabeta-dq 1/3(ph)
  Gain4/1 -> albe-dq/3(ph)
  albe-dq/2(vq) -> Out4/1
  Add4/1 -> Gain3/1
  abc-alphabeta 1/2(vbeta) -> k=0.1/1(u)
  Gain3/1 -> albe-dq/2(vbeta)
  abc-alphabeta 1/1(valpha) -> k=0.4/1(u)

== system node23_case_10kV_withLoad_v2/IBR-12/IBR1输出电流正负序分离 ==
  In1 : Inport
  Add1 : Sum  Inputs=+-
  Add2 : Sum
  Add3 : Sum
  Add4 : Sum  Inputs=+-
  Demux2 : Demux  Outputs=3
  Gain{,1..3} (4 alike) : Gain  Gain=0.5
  Gain4 : Gain  Gain=-1
  abc-alphabeta 1 : MATLAB Function  TreatAsAtomicUnit=on
  albe-dq : MATLAB Function  TreatAsAtomicUnit=on
  alphabeta-dq 1 : MATLAB Function  TreatAsAtomicUnit=on
  k=0.1 : Subsystem
  k=0.4 : Subsystem
  d+ : Outport  VectorParamsAs1DForOutWhenUnconnected=off
  q+ : Outport  Port=2  VectorParamsAs1DForOutWhenUnconnected=off
  d- : Outport  Port=3  VectorParamsAs1DForOutWhenUnconnected=off
  q- : Outport  Port=4  VectorParamsAs1DForOutWhenUnconnected=off
  wires:
  albe-dq/2(vq) -> q-/1
  albe-dq/1(vd) -> d-/1
  alphabeta-dq 1/2(vq) -> q+/1
  alphabeta-dq 1/1(vd) -> d+/1
  abc-alphabeta 1/1(valpha) -> k=0.4/1(u)
  Gain3/1 -> albe-dq/2(vbeta)
  abc-alphabeta 1/2(vbeta) -> k=0.1/1(u)
  Add4/1 -> Gain3/1
  Gain4/1 -> albe-dq/3(ph)
  [wt12] -> alphabeta-dq 1/3(ph)
  Demux2/3 -> abc-alphabeta 1/3(vc)
  Gain2/1 -> albe-dq/1(valpha)
  In1/1 -> Demux2/1
  Gain1/1 -> alphabeta-dq 1/2(vbeta)
  [wt12] -> Gain4/1
  Add3/1 -> Gain2/1
  Add2/1 -> Gain1/1
  k=0.1/2(qu') -> Add3/2, Add1/2
  k=0.4/2(qu') -> Add4/2, Add2/1
  Gain/1 -> alphabeta-dq 1/1(valpha)
  Demux2/1 -> abc-alphabeta 1/1(va)
  Add1/1 -> Gain/1
  k=0.1/1(u') -> Add2/2, Add4/1
  k=0.4/1(u') -> Add1/1, Add3/1
  Demux2/2 -> abc-alphabeta 1/2(vb)

== system node23_case_10kV_withLoad_v2/IBR-12/SOGI ==
  u : Inport
  Gain1 : Gain  Gain=314.15926
  Gain2 : Gain  Gain=0.707
  Gain3 : Gain  Gain=314.15926
  Integrator : Integrator
  Integrator1 : Integrator
  Sum : Sum  Inputs=-+|
  Sum1 : Sum  Inputs=|+-
  u' : Outport
  qu' : Outport  Port=2
  wires:
  Sum/1 -> Gain2/1
  Gain3/1 -> Sum1/2, qu'/1  "qu'"
  Integrator1/1 -> Gain3/1
  Gain2/1 -> Sum1/1
  Integrator/1 -> Sum/1, u'/1, Integrator1/1  "u'"
  u/1 -> Sum/2
  Sum1/1 -> Gain1/1
  Gain1/1 -> Integrator/1

== system node23_case_10kV_withLoad_v2/IBR-12/k=0.3 ==
  u : Inport
  Gain1 : Gain  Gain=314.15926
  Gain2 : Gain  Gain=0.707
  Gain3 : Gain  Gain=314.15926
  Integrator : Integrator
  Integrator1 : Integrator
  Sum : Sum  Inputs=-+|
  Sum1 : Sum  Inputs=|+-
  u' : Outport
  qu' : Outport  Port=2
  wires:
  Sum/1 -> Gain2/1
  Gain3/1 -> Sum1/2, qu'/1  "qu'"
  Integrator1/1 -> Gain3/1
  Gain2/1 -> Sum1/1
  Integrator/1 -> Sum/1, u'/1, Integrator1/1  "u'"
  u/1 -> Sum/2
  Sum1/1 -> Gain1/1
  Gain1/1 -> Integrator/1

== system node23_case_10kV_withLoad_v2/IBR-16/IBR1输出电压正负序分离 ==
  In1 : Inport
  Add1 : Sum  Inputs=+-
  Add2 : Sum
  Add3 : Sum
  Add4 : Sum  Inputs=+-
  Demux2 : Demux  Outputs=3
  Gain{,1..3} (4 alike) : Gain  Gain=0.5
  Gain4 : Gain  Gain=-1
  abc-alphabeta 1 : MATLAB Function  TreatAsAtomicUnit=on
  albe-dq : MATLAB Function  TreatAsAtomicUnit=on
  alphabeta-dq 1 : MATLAB Function  TreatAsAtomicUnit=on
  k=0.1 : Subsystem
  k=0.4 : Subsystem
  Out1 : Outport  VectorParamsAs1DForOutWhenUnconnected=off
  Out2 : Outport  Port=2  VectorParamsAs1DForOutWhenUnconnected=off
  Out3 : Outport  Port=3  VectorParamsAs1DForOutWhenUnconnected=off
  Out4 : Outport  Port=4  VectorParamsAs1DForOutWhenUnconnected=off
  wires:
  Demux2/2 -> abc-alphabeta 1/2(vb)
  k=0.4/1(u') -> Add3/1, Add1/1
  k=0.1/1(u') -> Add4/1, Add2/2
  Add1/1 -> Gain/1
  Demux2/1 -> abc-alphabeta 1/1(va)
  Gain/1 -> alphabeta-dq 1/1(valpha)
  k=0.4/2(qu') -> Add2/1, Add4/2
  albe-dq/1(vd) -> Out3/1
  k=0.1/2(qu') -> Add1/2, Add3/2
  Add2/1 -> Gain1/1
  alphabeta-dq 1/1(vd) -> Out1/1
  Add3/1 -> Gain2/1
  [wt16] -> Gain4/1
  Gain1/1 -> alphabeta-dq 1/2(vbeta)
  In1/1 -> Demux2/1
  Gain2/1 -> albe-dq/1(valpha)
  alphabeta-dq 1/2(vq) -> Out2/1
  Demux2/3 -> abc-alphabeta 1/3(vc)
  [wt16] -> alphabeta-dq 1/3(ph)
  Gain4/1 -> albe-dq/3(ph)
  albe-dq/2(vq) -> Out4/1
  Add4/1 -> Gain3/1
  abc-alphabeta 1/2(vbeta) -> k=0.1/1(u)
  Gain3/1 -> albe-dq/2(vbeta)
  abc-alphabeta 1/1(valpha) -> k=0.4/1(u)

== system node23_case_10kV_withLoad_v2/IBR-16/IBR1输出电流正负序分离 ==
  In1 : Inport
  Add1 : Sum  Inputs=+-
  Add2 : Sum
  Add3 : Sum
  Add4 : Sum  Inputs=+-
  Demux2 : Demux  Outputs=3
  Gain{,1..3} (4 alike) : Gain  Gain=0.5
  Gain4 : Gain  Gain=-1
  abc-alphabeta 1 : MATLAB Function  TreatAsAtomicUnit=on
  albe-dq : MATLAB Function  TreatAsAtomicUnit=on
  alphabeta-dq 1 : MATLAB Function  TreatAsAtomicUnit=on
  k=0.1 : Subsystem
  k=0.4 : Subsystem
  d+ : Outport  VectorParamsAs1DForOutWhenUnconnected=off
  q+ : Outport  Port=2  VectorParamsAs1DForOutWhenUnconnected=off
  d- : Outport  Port=3  VectorParamsAs1DForOutWhenUnconnected=off
  q- : Outport  Port=4  VectorParamsAs1DForOutWhenUnconnected=off
  wires:
  albe-dq/2(vq) -> q-/1
  albe-dq/1(vd) -> d-/1
  alphabeta-dq 1/2(vq) -> q+/1
  alphabeta-dq 1/1(vd) -> d+/1
  abc-alphabeta 1/1(valpha) -> k=0.4/1(u)
  Gain3/1 -> albe-dq/2(vbeta)
  abc-alphabeta 1/2(vbeta) -> k=0.1/1(u)
  Add4/1 -> Gain3/1
  Gain4/1 -> albe-dq/3(ph)
  [wt16] -> alphabeta-dq 1/3(ph)
  Demux2/3 -> abc-alphabeta 1/3(vc)
  Gain2/1 -> albe-dq/1(valpha)
  In1/1 -> Demux2/1
  Gain1/1 -> alphabeta-dq 1/2(vbeta)
  [wt16] -> Gain4/1
  Add3/1 -> Gain2/1
  Add2/1 -> Gain1/1
  k=0.1/2(qu') -> Add3/2, Add1/2
  k=0.4/2(qu') -> Add4/2, Add2/1
  Gain/1 -> alphabeta-dq 1/1(valpha)
  Demux2/1 -> abc-alphabeta 1/1(va)
  Add1/1 -> Gain/1
  k=0.1/1(u') -> Add2/2, Add4/1
  k=0.4/1(u') -> Add1/1, Add3/1
  Demux2/2 -> abc-alphabeta 1/2(vb)

== system node23_case_10kV_withLoad_v2/IBR-16/SOGI ==
  u : Inport
  Gain1 : Gain  Gain=314.15926
  Gain2 : Gain  Gain=0.707
  Gain3 : Gain  Gain=314.15926
  Integrator : Integrator
  Integrator1 : Integrator
  Sum : Sum  Inputs=-+|
  Sum1 : Sum  Inputs=|+-
  u' : Outport
  qu' : Outport  Port=2
  wires:
  Sum/1 -> Gain2/1
  Gain3/1 -> Sum1/2, qu'/1  "qu'"
  Integrator1/1 -> Gain3/1
  Gain2/1 -> Sum1/1
  Integrator/1 -> Sum/1, u'/1, Integrator1/1  "u'"
  u/1 -> Sum/2
  Sum1/1 -> Gain1/1
  Gain1/1 -> Integrator/1

== system node23_case_10kV_withLoad_v2/IBR-16/k=0.3 ==
  u : Inport
  Gain1 : Gain  Gain=314.15926
  Gain2 : Gain  Gain=0.707
  Gain3 : Gain  Gain=314.15926
  Integrator : Integrator
  Integrator1 : Integrator
  Sum : Sum  Inputs=-+|
  Sum1 : Sum  Inputs=|+-
  u' : Outport
  qu' : Outport  Port=2
  wires:
  Sum/1 -> Gain2/1
  Gain3/1 -> Sum1/2, qu'/1  "qu'"
  Integrator1/1 -> Gain3/1
  Gain2/1 -> Sum1/1
  Integrator/1 -> Sum/1, u'/1, Integrator1/1  "u'"
  u/1 -> Sum/2
  Sum1/1 -> Gain1/1
  Gain1/1 -> Integrator/1

== system node23_case_10kV_withLoad_v2/IBR-21/IBR1输出电压正负序分离 ==
  In1 : Inport
  Add1 : Sum  Inputs=+-
  Add2 : Sum
  Add3 : Sum
  Add4 : Sum  Inputs=+-
  Demux2 : Demux  Outputs=3
  Gain{,1..3} (4 alike) : Gain  Gain=0.5
  Gain4 : Gain  Gain=-1
  abc-alphabeta 1 : MATLAB Function  TreatAsAtomicUnit=on
  albe-dq : MATLAB Function  TreatAsAtomicUnit=on
  alphabeta-dq 1 : MATLAB Function  TreatAsAtomicUnit=on
  k=0.1 : Subsystem
  k=0.4 : Subsystem
  Out1 : Outport  VectorParamsAs1DForOutWhenUnconnected=off
  Out2 : Outport  Port=2  VectorParamsAs1DForOutWhenUnconnected=off
  Out3 : Outport  Port=3  VectorParamsAs1DForOutWhenUnconnected=off
  Out4 : Outport  Port=4  VectorParamsAs1DForOutWhenUnconnected=off
  wires:
  Demux2/2 -> abc-alphabeta 1/2(vb)
  k=0.4/1(u') -> Add3/1, Add1/1
  k=0.1/1(u') -> Add4/1, Add2/2
  Add1/1 -> Gain/1
  Demux2/1 -> abc-alphabeta 1/1(va)
  Gain/1 -> alphabeta-dq 1/1(valpha)
  k=0.4/2(qu') -> Add2/1, Add4/2
  albe-dq/1(vd) -> Out3/1
  k=0.1/2(qu') -> Add1/2, Add3/2
  Add2/1 -> Gain1/1
  alphabeta-dq 1/1(vd) -> Out1/1
  Add3/1 -> Gain2/1
  [wt21] -> Gain4/1
  Gain1/1 -> alphabeta-dq 1/2(vbeta)
  In1/1 -> Demux2/1
  Gain2/1 -> albe-dq/1(valpha)
  alphabeta-dq 1/2(vq) -> Out2/1
  Demux2/3 -> abc-alphabeta 1/3(vc)
  [wt21] -> alphabeta-dq 1/3(ph)
  Gain4/1 -> albe-dq/3(ph)
  albe-dq/2(vq) -> Out4/1
  Add4/1 -> Gain3/1
  abc-alphabeta 1/2(vbeta) -> k=0.1/1(u)
  Gain3/1 -> albe-dq/2(vbeta)
  abc-alphabeta 1/1(valpha) -> k=0.4/1(u)

== system node23_case_10kV_withLoad_v2/IBR-21/IBR1输出电流正负序分离 ==
  In1 : Inport
  Add1 : Sum  Inputs=+-
  Add2 : Sum
  Add3 : Sum
  Add4 : Sum  Inputs=+-
  Demux2 : Demux  Outputs=3
  Gain{,1..3} (4 alike) : Gain  Gain=0.5
  Gain4 : Gain  Gain=-1
  abc-alphabeta 1 : MATLAB Function  TreatAsAtomicUnit=on
  albe-dq : MATLAB Function  TreatAsAtomicUnit=on
  alphabeta-dq 1 : MATLAB Function  TreatAsAtomicUnit=on
  k=0.1 : Subsystem
  k=0.4 : Subsystem
  d+ : Outport  VectorParamsAs1DForOutWhenUnconnected=off
  q+ : Outport  Port=2  VectorParamsAs1DForOutWhenUnconnected=off
  d- : Outport  Port=3  VectorParamsAs1DForOutWhenUnconnected=off
  q- : Outport  Port=4  VectorParamsAs1DForOutWhenUnconnected=off
  wires:
  albe-dq/2(vq) -> q-/1
  albe-dq/1(vd) -> d-/1
  alphabeta-dq 1/2(vq) -> q+/1
  alphabeta-dq 1/1(vd) -> d+/1
  abc-alphabeta 1/1(valpha) -> k=0.4/1(u)
  Gain3/1 -> albe-dq/2(vbeta)
  abc-alphabeta 1/2(vbeta) -> k=0.1/1(u)
  Add4/1 -> Gain3/1
  Gain4/1 -> albe-dq/3(ph)
  [wt21] -> alphabeta-dq 1/3(ph)
  Demux2/3 -> abc-alphabeta 1/3(vc)
  Gain2/1 -> albe-dq/1(valpha)
  In1/1 -> Demux2/1
  Gain1/1 -> alphabeta-dq 1/2(vbeta)
  [wt21] -> Gain4/1
  Add3/1 -> Gain2/1
  Add2/1 -> Gain1/1
  k=0.1/2(qu') -> Add3/2, Add1/2
  k=0.4/2(qu') -> Add4/2, Add2/1
  Gain/1 -> alphabeta-dq 1/1(valpha)
  Demux2/1 -> abc-alphabeta 1/1(va)
  Add1/1 -> Gain/1
  k=0.1/1(u') -> Add2/2, Add4/1
  k=0.4/1(u') -> Add1/1, Add3/1
  Demux2/2 -> abc-alphabeta 1/2(vb)

== system node23_case_10kV_withLoad_v2/IBR-21/SOGI ==
  u : Inport
  Gain1 : Gain  Gain=314.15926
  Gain2 : Gain  Gain=0.707
  Gain3 : Gain  Gain=314.15926
  Integrator : Integrator
  Integrator1 : Integrator
  Sum : Sum  Inputs=-+|
  Sum1 : Sum  Inputs=|+-
  u' : Outport
  qu' : Outport  Port=2
  wires:
  Sum/1 -> Gain2/1
  Gain3/1 -> Sum1/2, qu'/1  "qu'"
  Integrator1/1 -> Gain3/1
  Gain2/1 -> Sum1/1
  Integrator/1 -> Sum/1, u'/1, Integrator1/1  "u'"
  u/1 -> Sum/2
  Sum1/1 -> Gain1/1
  Gain1/1 -> Integrator/1

== system node23_case_10kV_withLoad_v2/IBR-21/k=0.3 ==
  u : Inport
  Gain1 : Gain  Gain=314.15926
  Gain2 : Gain  Gain=0.707
  Gain3 : Gain  Gain=314.15926
  Integrator : Integrator
  Integrator1 : Integrator
  Sum : Sum  Inputs=-+|
  Sum1 : Sum  Inputs=|+-
  u' : Outport
  qu' : Outport  Port=2
  wires:
  Sum/1 -> Gain2/1
  Gain3/1 -> Sum1/2, qu'/1  "qu'"
  Integrator1/1 -> Gain3/1
  Gain2/1 -> Sum1/1
  Integrator/1 -> Sum/1, u'/1, Integrator1/1  "u'"
  u/1 -> Sum/2
  Sum1/1 -> Gain1/1
  Gain1/1 -> Integrator/1

== system node23_case_10kV_withLoad_v2/IBR-22/IBR1输出电压正负序分离 ==
  In1 : Inport
  Add1 : Sum  Inputs=+-
  Add2 : Sum
  Add3 : Sum
  Add4 : Sum  Inputs=+-
  Demux2 : Demux  Outputs=3
  Gain{,1..3} (4 alike) : Gain  Gain=0.5
  Gain4 : Gain  Gain=-1
  abc-alphabeta 1 : MATLAB Function  TreatAsAtomicUnit=on
  albe-dq : MATLAB Function  TreatAsAtomicUnit=on
  alphabeta-dq 1 : MATLAB Function  TreatAsAtomicUnit=on
  k=0.1 : Subsystem
  k=0.4 : Subsystem
  Out1 : Outport  VectorParamsAs1DForOutWhenUnconnected=off
  Out2 : Outport  Port=2  VectorParamsAs1DForOutWhenUnconnected=off
  Out3 : Outport  Port=3  VectorParamsAs1DForOutWhenUnconnected=off
  Out4 : Outport  Port=4  VectorParamsAs1DForOutWhenUnconnected=off
  wires:
  Demux2/2 -> abc-alphabeta 1/2(vb)
  k=0.4/1(u') -> Add3/1, Add1/1
  k=0.1/1(u') -> Add4/1, Add2/2
  Add1/1 -> Gain/1
  Demux2/1 -> abc-alphabeta 1/1(va)
  Gain/1 -> alphabeta-dq 1/1(valpha)
  k=0.4/2(qu') -> Add2/1, Add4/2
  albe-dq/1(vd) -> Out3/1
  k=0.1/2(qu') -> Add1/2, Add3/2
  Add2/1 -> Gain1/1
  alphabeta-dq 1/1(vd) -> Out1/1
  Add3/1 -> Gain2/1
  [wt22] -> Gain4/1
  Gain1/1 -> alphabeta-dq 1/2(vbeta)
  In1/1 -> Demux2/1
  Gain2/1 -> albe-dq/1(valpha)
  alphabeta-dq 1/2(vq) -> Out2/1
  Demux2/3 -> abc-alphabeta 1/3(vc)
  [wt22] -> alphabeta-dq 1/3(ph)
  Gain4/1 -> albe-dq/3(ph)
  albe-dq/2(vq) -> Out4/1
  Add4/1 -> Gain3/1
  abc-alphabeta 1/2(vbeta) -> k=0.1/1(u)
  Gain3/1 -> albe-dq/2(vbeta)
  abc-alphabeta 1/1(valpha) -> k=0.4/1(u)

== system node23_case_10kV_withLoad_v2/IBR-22/IBR1输出电流正负序分离 ==
  In1 : Inport
  Add1 : Sum  Inputs=+-
  Add2 : Sum
  Add3 : Sum
  Add4 : Sum  Inputs=+-
  Demux2 : Demux  Outputs=3
  Gain{,1..3} (4 alike) : Gain  Gain=0.5
  Gain4 : Gain  Gain=-1
  abc-alphabeta 1 : MATLAB Function  TreatAsAtomicUnit=on
  albe-dq : MATLAB Function  TreatAsAtomicUnit=on
  alphabeta-dq 1 : MATLAB Function  TreatAsAtomicUnit=on
  k=0.1 : Subsystem
  k=0.4 : Subsystem
  d+ : Outport  VectorParamsAs1DForOutWhenUnconnected=off
  q+ : Outport  Port=2  VectorParamsAs1DForOutWhenUnconnected=off
  d- : Outport  Port=3  VectorParamsAs1DForOutWhenUnconnected=off
  q- : Outport  Port=4  VectorParamsAs1DForOutWhenUnconnected=off
  wires:
  albe-dq/2(vq) -> q-/1
  albe-dq/1(vd) -> d-/1
  alphabeta-dq 1/2(vq) -> q+/1
  alphabeta-dq 1/1(vd) -> d+/1
  abc-alphabeta 1/1(valpha) -> k=0.4/1(u)
  Gain3/1 -> albe-dq/2(vbeta)
  abc-alphabeta 1/2(vbeta) -> k=0.1/1(u)
  Add4/1 -> Gain3/1
  Gain4/1 -> albe-dq/3(ph)
  [wt22] -> alphabeta-dq 1/3(ph)
  Demux2/3 -> abc-alphabeta 1/3(vc)
  Gain2/1 -> albe-dq/1(valpha)
  In1/1 -> Demux2/1
  Gain1/1 -> alphabeta-dq 1/2(vbeta)
  [wt22] -> Gain4/1
  Add3/1 -> Gain2/1
  Add2/1 -> Gain1/1
  k=0.1/2(qu') -> Add3/2, Add1/2
  k=0.4/2(qu') -> Add4/2, Add2/1
  Gain/1 -> alphabeta-dq 1/1(valpha)
  Demux2/1 -> abc-alphabeta 1/1(va)
  Add1/1 -> Gain/1
  k=0.1/1(u') -> Add2/2, Add4/1
  k=0.4/1(u') -> Add1/1, Add3/1
  Demux2/2 -> abc-alphabeta 1/2(vb)

== system node23_case_10kV_withLoad_v2/IBR-22/SOGI ==
  u : Inport
  Gain1 : Gain  Gain=314.15926
  Gain2 : Gain  Gain=0.707
  Gain3 : Gain  Gain=314.15926
  Integrator : Integrator
  Integrator1 : Integrator
  Sum : Sum  Inputs=-+|
  Sum1 : Sum  Inputs=|+-
  u' : Outport
  qu' : Outport  Port=2
  wires:
  Sum/1 -> Gain2/1
  Gain3/1 -> Sum1/2, qu'/1  "qu'"
  Integrator1/1 -> Gain3/1
  Gain2/1 -> Sum1/1
  Integrator/1 -> Sum/1, u'/1, Integrator1/1  "u'"
  u/1 -> Sum/2
  Sum1/1 -> Gain1/1
  Gain1/1 -> Integrator/1

== system node23_case_10kV_withLoad_v2/IBR-22/k=0.3 ==
  u : Inport
  Gain1 : Gain  Gain=314.15926
  Gain2 : Gain  Gain=0.707
  Gain3 : Gain  Gain=314.15926
  Integrator : Integrator
  Integrator1 : Integrator
  Sum : Sum  Inputs=-+|
  Sum1 : Sum  Inputs=|+-
  u' : Outport
  qu' : Outport  Port=2
  wires:
  Sum/1 -> Gain2/1
  Gain3/1 -> Sum1/2, qu'/1  "qu'"
  Integrator1/1 -> Gain3/1
  Gain2/1 -> Sum1/1
  Integrator/1 -> Sum/1, u'/1, Integrator1/1  "u'"
  u/1 -> Sum/2
  Sum1/1 -> Gain1/1
  Gain1/1 -> Integrator/1

== system node23_case_10kV_withLoad_v2/IBR-23/IBR1输出电压正负序分离 ==
  In1 : Inport
  Add1 : Sum  Inputs=+-
  Add2 : Sum
  Add3 : Sum
  Add4 : Sum  Inputs=+-
  Demux2 : Demux  Outputs=3
  Gain{,1..3} (4 alike) : Gain  Gain=0.5
  Gain4 : Gain  Gain=-1
  abc-alphabeta 1 : MATLAB Function  TreatAsAtomicUnit=on
  albe-dq : MATLAB Function  TreatAsAtomicUnit=on
  alphabeta-dq 1 : MATLAB Function  TreatAsAtomicUnit=on
  k=0.1 : Subsystem
  k=0.4 : Subsystem
  Out1 : Outport  VectorParamsAs1DForOutWhenUnconnected=off
  Out2 : Outport  Port=2  VectorParamsAs1DForOutWhenUnconnected=off
  Out3 : Outport  Port=3  VectorParamsAs1DForOutWhenUnconnected=off
  Out4 : Outport  Port=4  VectorParamsAs1DForOutWhenUnconnected=off
  wires:
  Demux2/2 -> abc-alphabeta 1/2(vb)
  k=0.4/1(u') -> Add3/1, Add1/1
  k=0.1/1(u') -> Add4/1, Add2/2
  Add1/1 -> Gain/1
  Demux2/1 -> abc-alphabeta 1/1(va)
  Gain/1 -> alphabeta-dq 1/1(valpha)
  k=0.4/2(qu') -> Add2/1, Add4/2
  albe-dq/1(vd) -> Out3/1
  k=0.1/2(qu') -> Add1/2, Add3/2
  Add2/1 -> Gain1/1
  alphabeta-dq 1/1(vd) -> Out1/1
  Add3/1 -> Gain2/1
  [wt23] -> Gain4/1
  Gain1/1 -> alphabeta-dq 1/2(vbeta)
  In1/1 -> Demux2/1
  Gain2/1 -> albe-dq/1(valpha)
  alphabeta-dq 1/2(vq) -> Out2/1
  Demux2/3 -> abc-alphabeta 1/3(vc)
  [wt23] -> alphabeta-dq 1/3(ph)
  Gain4/1 -> albe-dq/3(ph)
  albe-dq/2(vq) -> Out4/1
  Add4/1 -> Gain3/1
  abc-alphabeta 1/2(vbeta) -> k=0.1/1(u)
  Gain3/1 -> albe-dq/2(vbeta)
  abc-alphabeta 1/1(valpha) -> k=0.4/1(u)

== system node23_case_10kV_withLoad_v2/IBR-23/IBR1输出电流正负序分离 ==
  In1 : Inport
  Add1 : Sum  Inputs=+-
  Add2 : Sum
  Add3 : Sum
  Add4 : Sum  Inputs=+-
  Demux2 : Demux  Outputs=3
  Gain{,1..3} (4 alike) : Gain  Gain=0.5
  Gain4 : Gain  Gain=-1
  abc-alphabeta 1 : MATLAB Function  TreatAsAtomicUnit=on
  albe-dq : MATLAB Function  TreatAsAtomicUnit=on
  alphabeta-dq 1 : MATLAB Function  TreatAsAtomicUnit=on
  k=0.1 : Subsystem
  k=0.4 : Subsystem
  d+ : Outport  VectorParamsAs1DForOutWhenUnconnected=off
  q+ : Outport  Port=2  VectorParamsAs1DForOutWhenUnconnected=off
  d- : Outport  Port=3  VectorParamsAs1DForOutWhenUnconnected=off
  q- : Outport  Port=4  VectorParamsAs1DForOutWhenUnconnected=off
  wires:
  albe-dq/2(vq) -> q-/1
  albe-dq/1(vd) -> d-/1
  alphabeta-dq 1/2(vq) -> q+/1
  alphabeta-dq 1/1(vd) -> d+/1
  abc-alphabeta 1/1(valpha) -> k=0.4/1(u)
  Gain3/1 -> albe-dq/2(vbeta)
  abc-alphabeta 1/2(vbeta) -> k=0.1/1(u)
  Add4/1 -> Gain3/1
  Gain4/1 -> albe-dq/3(ph)
  [wt23] -> alphabeta-dq 1/3(ph)
  Demux2/3 -> abc-alphabeta 1/3(vc)
  Gain2/1 -> albe-dq/1(valpha)
  In1/1 -> Demux2/1
  Gain1/1 -> alphabeta-dq 1/2(vbeta)
  [wt23] -> Gain4/1
  Add3/1 -> Gain2/1
  Add2/1 -> Gain1/1
  k=0.1/2(qu') -> Add3/2, Add1/2
  k=0.4/2(qu') -> Add4/2, Add2/1
  Gain/1 -> alphabeta-dq 1/1(valpha)
  Demux2/1 -> abc-alphabeta 1/1(va)
  Add1/1 -> Gain/1
  k=0.1/1(u') -> Add2/2, Add4/1
  k=0.4/1(u') -> Add1/1, Add3/1
  Demux2/2 -> abc-alphabeta 1/2(vb)
